simulink model "BLDC_SMC"  (R2023b)
settings: Solver=ode23tb  StartTime=0.0  StopTime=2  FixedStep=Ts  RelTol=1e-4  EnableMultiTasking=on
InitFcn:
  | Ts = 10e-6;
  | 
  | R = 2.875;
  | Ld = 8.2e-3;
  | Lq = 8.2e-3;
  | Pn = 4;
  | flux = 0.175;
model workspace (MAT data in the model file):
  LDLQ = [0.00108 0.00108]
  PN_ = 7
  RS = 4.64
  TS_1 = 0.001
undefined symbols (not defined in the file): DiscIntNeverNeededParam
libraries: simulink x14, powerlib_extras x12, spsPermanentMagnetSynchronousMachineLib x6, spsUniversalBridgeLib x6, spsDCVoltageSourceLib x6, sps_lib x6, dspindex x2, visionanalysis x1, dspstat3 x1, dspfdesign x1
(part 1 of 3)
settings Model: PacingRate=100  Creator=SUN  LastModifiedBy=Shykerboy
settings SolverCC: ZeroCrossControl=DisableAll  AlgebraicLoopSolver=TrustRegion
settings DataIOCC: LimitDataPoints=on  SaveFormat=Array  SignalLoggingSaveFormat=ModelDataLogs  ReturnWorkspaceOutputs=off
settings OptimizationCC: ExpressionDepthLimit=2147483647  InitFltsAndDblsToZero=on  LifeSpan=inf
settings DebuggingCC: UnderspecifiedInitializationDetection=Classic  MergeDetectMultiDrivingBlocksExec=none  SolverPrmCheckMsg=warning  FcnCallInpInsideContextMsg=warning  UnconnectedInputMsg=warning  UnconnectedOutputMsg=warning  UnconnectedLineMsg=warning  StateNameClashWarn=warning  SFUnexpectedBacktrackingDiag=warning  SFNoUnconditionalDefaultTransitionDiag=warning  SFExecutionAtInitializationDiag=none  ArithmeticOperatorsInVariantConditions=warning
settings HardwareCC: ProdBitPerPointer=32  ProdBitPerSizeT=32  ProdBitPerPtrDiffT=32  ProdLargestAtomicFloat=None  ProdIntDivRoundTo=Undefined  ProdEndianess=Unspecified  ProdWordSize=32  ProdHWDeviceType=32-bit Generic
settings ModelReferenceCC: PropagateSignalLabelsOutOfModel=off
settings SFSimCC: SimUseLocalCustomCode=off  CustomCodeUndefinedFunction=UseInterfaceOnly
settings RTWCC: RTWUseLocalCustomCode=off
settings CodeAppCC: StateflowObjectComments=on
settings GRTTargetCC: TargetLangStandard=C89/C90 (ANSI)  CombineOutputUpdateFcns=off  GRTInterface=on
settings ConfigComp: CovMetricSettings=dw  CovSaveCumulativeToWorkspaceVar=on  CovSaveSingleToWorkspaceVar=on  CovExternalEMLEnable=off  CovSFcnEnable=off
settings SimscapeCC: SimscapeNormalizeSystem=off

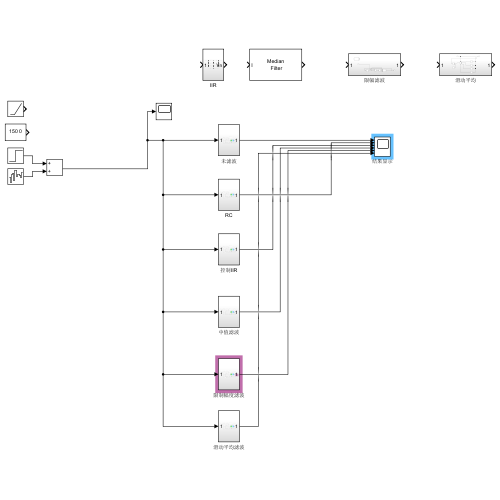
[thumbnail: Simulink's stored preview of the top-level diagram]
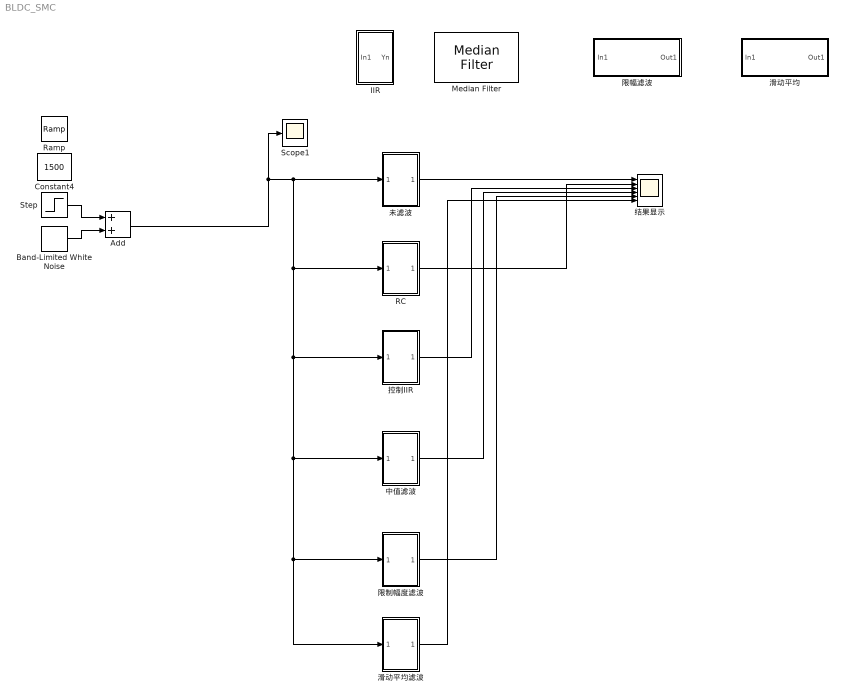
== system BLDC_SMC ==
  Add : Sum
  Band-Limited White Noise : simulink/Sources/Band-Limited White Noise  Cov=[0.100]  Ts=0.001  seed=[23341]
  Constant4 : Constant  Value=1500  SampleTime=1e-3
  IIR : Subsystem
  Median Filter : visionanalysis/Median Filter  nghbood=[3 3]  outSize=Same as input port I  padType=Constant  padSrc=Specify via dialog  padVal=0  roundingMode=Floor  overflowMode=off
  RC : Subsystem
  Ramp : simulink/Sources/Ramp  slope=500  start=0  InitialOutput=0
  Scope1 : Scope
  Step : Step  Time=0.5  After=1000  SampleTime=1e-3
  中值滤波 : Subsystem
  控制IIR : Subsystem
  未滤波 : Subsystem
  滑动平均 : Subsystem
  滑动平均滤波 : Subsystem
  结果显示 : Scope  NumInputPorts=6
  限制幅度滤波 : Subsystem
  限幅滤波 : Subsystem
  wires:
  未滤波/1(Out1) -> 结果显示/1
  Step/1 -> Add/1
  Band-Limited White Noise/1 -> Add/2
  Add/1 -> Scope1/1, 滑动平均滤波/1(In1), 限制幅度滤波/1(In1), 中值滤波/1(In1), 控制IIR/1(In1), RC/1(In1), 未滤波/1(In1)
  RC/1(Out1) -> 结果显示/2
  控制IIR/1(Out1) -> 结果显示/3
  中值滤波/1(Out1) -> 结果显示/4
  限制幅度滤波/1(Out1) -> 结果显示/5
  滑动平均滤波/1(Out1) -> 结果显示/6

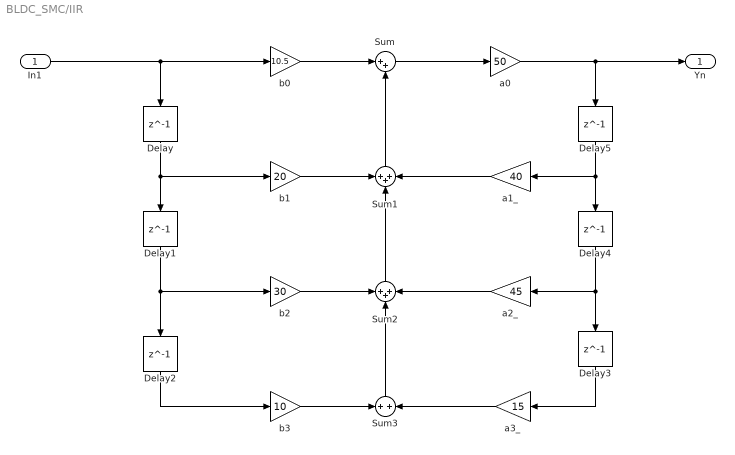
== system BLDC_SMC/IIR ==
  In1 : Inport
  Delay{,1..5} (6 alike) : Delay  DelayLength=1
  Sum : Sum  Inputs=|++
  Sum1 : Sum  Inputs=+++
  Sum2 : Sum  Inputs=+++
  Sum3 : Sum  Inputs=+|+
  a0 : Gain  Gain=50
  a1_ : Gain  Gain=40
  a2_ : Gain  Gain=45
  a3_ : Gain  Gain=15
  b0 : Gain  Gain=10.5
  b1 : Gain  Gain=20
  b2 : Gain  Gain=30
  b3 : Gain  Gain=10
  Yn : Outport
  wires:
  Delay5/1 -> a1_/1, Delay4/1
  Sum2/1 -> Sum1/2
  Delay/1 -> b1/1, Delay1/1
  a3_/1 -> Sum3/2
  Delay1/1 -> b2/1, Delay2/1
  b1/1 -> Sum1/1
  Delay3/1 -> a3_/1
  a0/1 -> Yn/1, Delay5/1
  b3/1 -> Sum3/1
  Delay4/1 -> a2_/1, Delay3/1
  b0/1 -> Sum/1
  a2_/1 -> Sum2/3
  Sum3/1 -> Sum2/2
  a1_/1 -> Sum1/3
  Sum1/1 -> Sum/2
  Delay2/1 -> b3/1
  b2/1 -> Sum2/1
  Sum/1 -> a0/1
  In1/1 -> b0/1, Delay/1

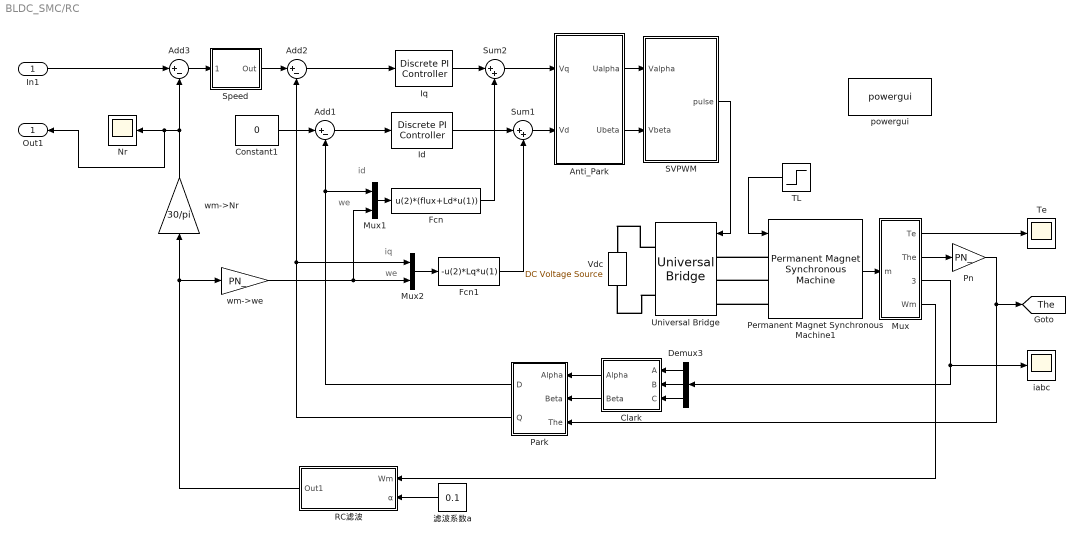
== system BLDC_SMC/RC ==
  note: iq
  note: we
  note: we
  note: id
  In1 : Inport
  Add1 : Sum  Inputs=|+-
  Add2 : Sum  Inputs=|+-
  Add3 : Sum  Inputs=|+-
  Anti_Park : Subsystem
  Clark : Subsystem
  Constant1 : Constant  Value=0
  Demux3 : Demux  Outputs=3
  Fcn : Fcn  Expr=u(2)*(flux+Ld*u(1))
  Fcn1 : Fcn  Expr=-u(2)*Lq*u(1)
  Id : powerlib_extras/Discrete  Control Blocks/Discrete PI Controller  Kp=Ld*2000  Ki=RS*2000  Par_Limits=[311*0.9*sqrt(1/3) -311*0.9*sqrt(1/3)]  Init=0  Ts=TS_1
  Iq : powerlib_extras/Discrete  Control Blocks/Discrete PI Controller  Kp=Lq*2000  Ki=RS*2000  Par_Limits=[311*0.9*sqrt(1/3) -311*0.9*sqrt(1/3)]  Init=0  Ts=TS_1
  Mux : Subsystem
  Mux1 : Mux  Inputs=2
  Mux2 : Mux  Inputs=2
  Nr : Scope
  Park : Subsystem
  Permanent Magnet Synchronous Machine1 : spsPermanentMagnetSynchronousMachineLib/Permanent Magnet Synchronous Machine  NbPhases=3  FluxDistribution=Sinusoidal  RotorType=Salient-pole  MechanicalLoad=Torque Tm  PresetModel=No  ShowDetailedParameters=on  MeasurementBus=off  Resistance=RS  Inductance=8.5e-3  dqInductances=LDLQ  La=0.000835  MachineConstant=Flux linkage established by magnets (V.s)  Flux=0.175  VoltageCst=222.1904  TorqueCst=1.8375  Flat=120  Mechanical=[0.003 0.008 7 0]  PolePairs=3  InitialConditions=[0,0, 0,0]  InitialConditions5ph=[0 0 0 0 0 0]  RefAngle=Aligned with phase A axis (original Park)  IterativeDiscreteModel=Trapezoidal non iterative  TsBlock=-1  TsPowergui=0
  Pn : Gain  Gain=PN_
  RC滤波 : Subsystem
  SVPWM : Subsystem
  Speed : Subsystem  AncestorBlock=|  DialogController=POWERSYS.PowerSysDialog  mask(Discrete PI Controller){C=60, Mu=200, q=300, Par_Limits=[30 -30], Init=0, Ts=TS_1}
      | powerlib_extras/Discrete 
      | Control Blocks/Discrete
      | PI Controller
      mask prompts: C "Gain (c):"; Mu "Gain (Mu):"; q "Gain (q)"; Par_Limits "Output limits: [ Upper   Lower ]"; Init "Output initial value:"; Ts "Sample time:"
      mask help: This block implements a discrete PI controller.
      mask init:
      | UpperLimit=Par_Limits(1);
      | LowerLimit=Par_Limits(2);
      | power_initmask();
      mask Help: This block is part of a subset of blocks in the Extras library that does not have documentation associated with it, other than the block mask description.
      mask Display: disp('SMC');
  Sum1 : Sum  Inputs=|++
  Sum2 : Sum  Inputs=|++
  TL : Step  Time=0.2  After=10  SampleTime=0
  Te : Scope
  Universal Bridge : spsUniversalBridgeLib/Universal Bridge  Arms=3  SnubberResistance=1e5  SnubberCapacitance=inf  Device=IGBT / Diodes  Ron=1e-3  Lon=0  ForwardVoltages="[  0  0  ]"  ForwardVoltage=0  GTOparameters=[ 10e-6 , 20e-6 ]  IGBTparameters=[ 1e-6 , 2e-6 ]  Measurements=None  Measurements_2=None  converterType=Rectifier
  Vdc : spsDCVoltageSourceLib/DC Voltage Source  Amplitude=311  Measurements=None
  iabc : Scope
  powergui : sps_lib/powergui  SimulationMode=Continuous  SampleTime=Ts  frequency=60  Iterations=50  frequencyindice=0  Pbase=100e6  ErrMax=1e-4  UnitsV=kV  UnitsW=MW  buscounter=0  FunctionMessages=off  echomessages=off  EnableUseOfTLC=off  CurrentSourceSwitches=on  DisableSnubberDevices=off  DisableRonSwitches=off  DisableVfSwitches=off  DisplayEquations=off  AutomaticDiscreteSolvers=off  SolverType=Tustin/Backward Euler (TBE)  Interpol=off  ExternalGateDelay=off  methode=off  Ts=0  x0status=blocks  SPID=off  SwTol=0  HookPort=off  NonlinearTolerance=1e-4  nMaxIteration=100  ContinueOnMaxIteration=off  RestoreLinks=warning  ResistiveCurrentMeasurement=off  Frange=[0:2:500]  Ylog=off  Xlog=on  ShowGrid=off  save=off  variable=ZData  structure=0  ZoomFFT=on  StartTime=0.0  cycles=1  DisplayStyle=1  fundamental=60  FreqAxis=off  MaxFrequency=1000  frequencyindicesteady=1  RmsSteady=1  display=off
  wm->Nr : Gain  Gain=30/pi
  wm->we : Gain  Gain=PN_
  滤波系数a : Constant  Value=0.1
  Out1 : Outport
  tag scope: The=global
  wires:
  Pn/1 -> Park/3(The), [The]
  SVPWM/1(pulse) -> Universal Bridge/1
  Add1/1 -> Id/1
  In1/1 -> Add3/1
  Fcn/1 -> Sum2/2
  Id/1 -> Sum1/1
  Mux2/1 -> Fcn1/1
  wm->Nr/1 -> Add3/2, Out1/1, Nr/1
  Clark/2(Beta) -> Park/2(Beta)
  Iq/1 -> Sum2/1
  Sum2/1 -> Anti_Park/1(Vq)
  Speed/1(Out) -> Add2/1
  Add2/1 -> Iq/1
  Fcn1/1 -> Sum1/2
  Park/2(Q) -> Mux2/1, Add2/2
  Constant1/1 -> Add1/1
  Sum1/1 -> Anti_Park/2(Vd)
  Add3/1 -> Speed/1(Error)
  Mux/1(Te) -> Te/1
  Mux/2(The) -> Pn/1
  Anti_Park/2(Ubeta) -> SVPWM/2(Vbeta)
  Demux3/1 -> Clark/1(A)
  Demux3/3 -> Clark/3(C)
  Mux/3(Iabc) -> iabc/1, Demux3/1
  Demux3/2 -> Clark/2(B)
  Mux1/1 -> Fcn/1
  TL/1 -> Permanent Magnet Synchronous Machine1/1
  Permanent Magnet Synchronous Machine1/1 -> Mux/1(m)
  Clark/1(Alpha) -> Park/1(Alpha)
  Park/1(D) -> Mux1/1, Add1/2
  Anti_Park/1(Ualpha) -> SVPWM/1(Valpha)
  wm->we/1 -> Mux2/2, Mux1/2
  Mux/4(Wm) -> RC滤波/1(Wm)
  滤波系数a/1 -> RC滤波/2(α)
  RC滤波/1(Out1) -> wm->we/1, wm->Nr/1
  connections:
  Permanent Magnet Synchronous Machine1/LConn2 -- Universal Bridge/LConn2
  Universal Bridge/RConn1 -- Vdc/RConn1
  Permanent Magnet Synchronous Machine1/LConn1 -- Universal Bridge/LConn1
  Permanent Magnet Synchronous Machine1/LConn3 -- Universal Bridge/LConn3
  Universal Bridge/RConn2 -- Vdc/LConn1

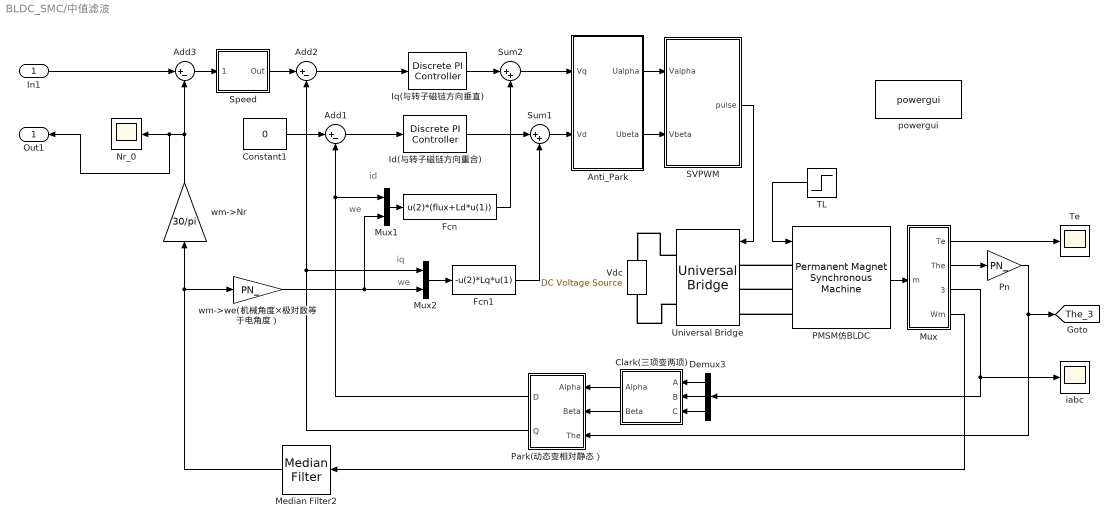
== system BLDC_SMC/中值滤波 ==
  note: iq
  note: we
  note: we
  note: id
  In1 : Inport
  Add1 : Sum  Inputs=|+-
  Add2 : Sum  Inputs=|+-
  Add3 : Sum  Inputs=|+-
  Anti_Park : Subsystem
  Clark(三项变两项) : Subsystem
  Constant1 : Constant  Value=0
  Demux3 : Demux  Outputs=3
  Fcn : Fcn  Expr=u(2)*(flux+Ld*u(1))
  Fcn1 : Fcn  Expr=-u(2)*Lq*u(1)
  Id(与转子磁链方向重合) : powerlib_extras/Discrete  Control Blocks/Discrete PI Controller  Kp=Ld*2000  Ki=RS*2000  Par_Limits=[311*0.9*sqrt(1/3) -311*0.9*sqrt(1/3)]  Init=0  Ts=TS_1
  Iq(与转子磁链方向垂直) : powerlib_extras/Discrete  Control Blocks/Discrete PI Controller  Kp=Lq*2000  Ki=RS*2000  Par_Limits=[311*0.9*sqrt(1/3) -311*0.9*sqrt(1/3)]  Init=0  Ts=TS_1
  Median Filter2 : dspstat3/Median Filter  WindowLength=5  SimulateUsing=Code generation
  Mux : Subsystem
  Mux1 : Mux  Inputs=2
  Mux2 : Mux  Inputs=2
  Nr_0 : Scope
  PMSM仿BLDC : spsPermanentMagnetSynchronousMachineLib/Permanent Magnet Synchronous Machine  NbPhases=3  FluxDistribution=Sinusoidal  RotorType=Salient-pole  MechanicalLoad=Torque Tm  PresetModel=No  ShowDetailedParameters=on  MeasurementBus=off  Resistance=RS  Inductance=8.5e-3  dqInductances=LDLQ  La=0.000835  MachineConstant=Flux linkage established by magnets (V.s)  Flux=0.175  VoltageCst=222.1904  TorqueCst=1.8375  Flat=120  Mechanical=[0.003 0.008 7 0]  PolePairs=3  InitialConditions=[0,0, 0,0]  InitialConditions5ph=[0 0 0 0 0 0]  RefAngle=Aligned with phase A axis (original Park)  IterativeDiscreteModel=Trapezoidal non iterative  TsBlock=-1  TsPowergui=0
  Park(动态变相对静态） : Subsystem
  Pn : Gain  Gain=PN_
  SVPWM : Subsystem
  Speed : Subsystem  AncestorBlock=|  DialogController=POWERSYS.PowerSysDialog  mask(Discrete PI Controller){C=60, Mu=200, q=300, Par_Limits=[30 -30], Init=0, Ts=TS_1}
      | powerlib_extras/Discrete 
      | Control Blocks/Discrete
      | PI Controller
      mask prompts: C "Gain (c):"; Mu "Gain (Mu):"; q "Gain (q)"; Par_Limits "Output limits: [ Upper   Lower ]"; Init "Output initial value:"; Ts "Sample time:"
      mask help: This block implements a discrete PI controller.
      mask init:
      | UpperLimit=Par_Limits(1);
      | LowerLimit=Par_Limits(2);
      | power_initmask();
      mask Help: This block is part of a subset of blocks in the Extras library that does not have documentation associated with it, other than the block mask description.
      mask Display: disp('SMC');
  Sum1 : Sum  Inputs=|++
  Sum2 : Sum  Inputs=|++
  TL : Step  Time=0.2  After=10  SampleTime=0
  Te : Scope
  Universal Bridge : spsUniversalBridgeLib/Universal Bridge  Arms=3  SnubberResistance=1e5  SnubberCapacitance=inf  Device=IGBT / Diodes  Ron=1e-3  Lon=0  ForwardVoltages="[  0  0  ]"  ForwardVoltage=0  GTOparameters=[ 10e-6 , 20e-6 ]  IGBTparameters=[ 1e-6 , 2e-6 ]  Measurements=None  Measurements_2=None  converterType=Rectifier
  Vdc : spsDCVoltageSourceLib/DC Voltage Source  Amplitude=311  Measurements=None
  iabc : Scope
  powergui : sps_lib/powergui  SimulationMode=Continuous  SampleTime=Ts  frequency=60  Iterations=50  frequencyindice=0  Pbase=100e6  ErrMax=1e-4  UnitsV=kV  UnitsW=MW  buscounter=0  FunctionMessages=off  echomessages=off  EnableUseOfTLC=off  CurrentSourceSwitches=on  DisableSnubberDevices=off  DisableRonSwitches=off  DisableVfSwitches=off  DisplayEquations=off  AutomaticDiscreteSolvers=off  SolverType=Tustin/Backward Euler (TBE)  Interpol=off  ExternalGateDelay=off  methode=off  Ts=0  x0status=blocks  SPID=off  SwTol=0  HookPort=off  NonlinearTolerance=1e-4  nMaxIteration=100  ContinueOnMaxIteration=off  RestoreLinks=warning  ResistiveCurrentMeasurement=off  Frange=[0:2:500]  Ylog=off  Xlog=on  ShowGrid=off  save=off  variable=ZData  structure=0  ZoomFFT=on  StartTime=0.0  cycles=1  DisplayStyle=1  fundamental=60  FreqAxis=off  MaxFrequency=1000  frequencyindicesteady=1  RmsSteady=1  display=off
  wm->Nr : Gain  Gain=30/pi
  wm->we(机械角度×极对数等于电角度） : Gain  Gain=PN_
  Out1 : Outport
  tag scope: The_3=global
  wires:
  Pn/1 -> Park(动态变相对静态）/3(The), [The_3]
  SVPWM/1(pulse) -> Universal Bridge/1
  Add1/1 -> Id(与转子磁链方向重合)/1
  In1/1 -> Add3/1
  Fcn/1 -> Sum2/2
  Id(与转子磁链方向重合)/1 -> Sum1/1
  Mux2/1 -> Fcn1/1
  wm->Nr/1 -> Add3/2, Out1/1, Nr_0/1
  Clark(三项变两项)/2(Beta) -> Park(动态变相对静态）/2(Beta)
  Iq(与转子磁链方向垂直)/1 -> Sum2/1
  Sum2/1 -> Anti_Park/1(Vq)
  Speed/1(Out) -> Add2/1
  Add2/1 -> Iq(与转子磁链方向垂直)/1
  Fcn1/1 -> Sum1/2
  Park(动态变相对静态）/2(Q) -> Mux2/1, Add2/2
  Constant1/1 -> Add1/1
  Sum1/1 -> Anti_Park/2(Vd)
  Add3/1 -> Speed/1(Error)
  Mux/1(Te) -> Te/1
  Mux/2(The) -> Pn/1
  Anti_Park/2(Ubeta) -> SVPWM/2(Vbeta)
  Demux3/1 -> Clark(三项变两项)/1(A)
  Demux3/3 -> Clark(三项变两项)/3(C)
  Mux/3(Iabc) -> iabc/1, Demux3/1
  Demux3/2 -> Clark(三项变两项)/2(B)
  Mux1/1 -> Fcn/1
  TL/1 -> PMSM仿BLDC/1
  PMSM仿BLDC/1 -> Mux/1(m)
  Clark(三项变两项)/1(Alpha) -> Park(动态变相对静态）/1(Alpha)
  Park(动态变相对静态）/1(D) -> Mux1/1, Add1/2
  Anti_Park/1(Ualpha) -> SVPWM/1(Valpha)
  wm->we(机械角度×极对数等于电角度）/1 -> Mux2/2, Mux1/2
  Mux/4(Wm) -> Median Filter2/1
  Median Filter2/1 -> wm->Nr/1, wm->we(机械角度×极对数等于电角度）/1
  connections:
  PMSM仿BLDC/LConn2 -- Universal Bridge/LConn2
  Universal Bridge/RConn1 -- Vdc/RConn1
  PMSM仿BLDC/LConn1 -- Universal Bridge/LConn1
  PMSM仿BLDC/LConn3 -- Universal Bridge/LConn3
  Universal Bridge/RConn2 -- Vdc/LConn1

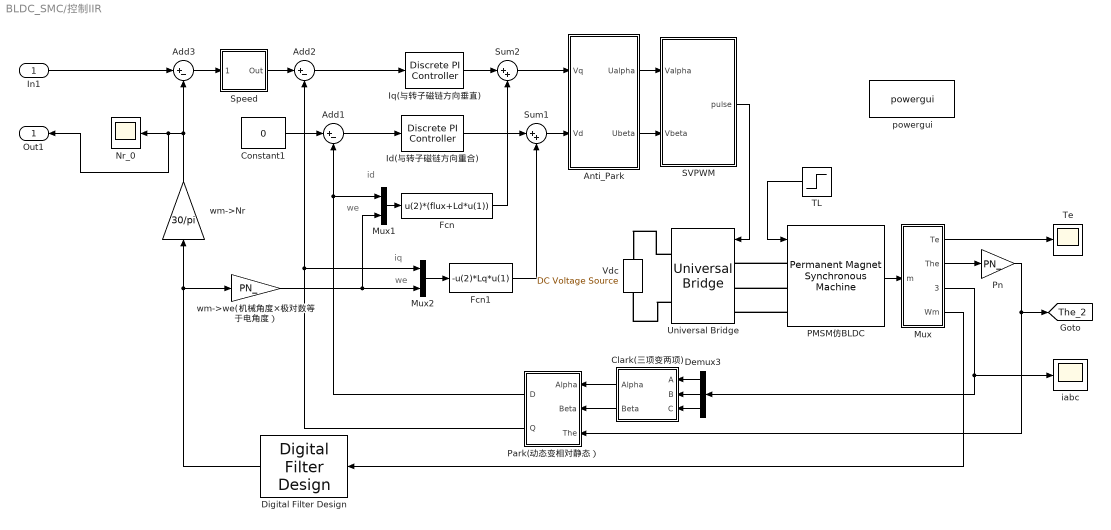
== system BLDC_SMC/控制IIR ==
  note: iq
  note: we
  note: we
  note: id
  In1 : Inport
  Add1 : Sum  Inputs=|+-
  Add2 : Sum  Inputs=|+-
  Add3 : Sum  Inputs=|+-
  Anti_Park : Subsystem
  Clark(三项变两项) : Subsystem
  Constant1 : Constant  Value=0
  Demux3 : Demux  Outputs=3
  Digital Filter Design : dspfdesign/Digital Filter Design  mwdsp_browser_bugfix_var=off
  Fcn : Fcn  Expr=u(2)*(flux+Ld*u(1))
  Fcn1 : Fcn  Expr=-u(2)*Lq*u(1)
  Id(与转子磁链方向重合) : powerlib_extras/Discrete  Control Blocks/Discrete PI Controller  Kp=Ld*2000  Ki=RS*2000  Par_Limits=[311*0.9*sqrt(1/3) -311*0.9*sqrt(1/3)]  Init=0  Ts=TS_1
  Iq(与转子磁链方向垂直) : powerlib_extras/Discrete  Control Blocks/Discrete PI Controller  Kp=Lq*2000  Ki=RS*2000  Par_Limits=[311*0.9*sqrt(1/3) -311*0.9*sqrt(1/3)]  Init=0  Ts=TS_1
  Mux : Subsystem
  Mux1 : Mux  Inputs=2
  Mux2 : Mux  Inputs=2
  Nr_0 : Scope
  PMSM仿BLDC : spsPermanentMagnetSynchronousMachineLib/Permanent Magnet Synchronous Machine  NbPhases=3  FluxDistribution=Sinusoidal  RotorType=Salient-pole  MechanicalLoad=Torque Tm  PresetModel=No  ShowDetailedParameters=on  MeasurementBus=off  Resistance=RS  Inductance=8.5e-3  dqInductances=LDLQ  La=0.000835  MachineConstant=Flux linkage established by magnets (V.s)  Flux=0.175  VoltageCst=222.1904  TorqueCst=1.8375  Flat=120  Mechanical=[0.003 0.008 7 0]  PolePairs=3  InitialConditions=[0,0, 0,0]  InitialConditions5ph=[0 0 0 0 0 0]  RefAngle=Aligned with phase A axis (original Park)  IterativeDiscreteModel=Trapezoidal non iterative  TsBlock=-1  TsPowergui=0
  Park(动态变相对静态） : Subsystem
  Pn : Gain  Gain=PN_
  SVPWM : Subsystem
  Speed : Subsystem  AncestorBlock=|  DialogController=POWERSYS.PowerSysDialog  mask(Discrete PI Controller){C=60, Mu=200, q=300, Par_Limits=[30 -30], Init=0, Ts=TS_1}
      | powerlib_extras/Discrete 
      | Control Blocks/Discrete
      | PI Controller
      mask prompts: C "Gain (c):"; Mu "Gain (Mu):"; q "Gain (q)"; Par_Limits "Output limits: [ Upper   Lower ]"; Init "Output initial value:"; Ts "Sample time:"
      mask help: This block implements a discrete PI controller.
      mask init:
      | UpperLimit=Par_Limits(1);
      | LowerLimit=Par_Limits(2);
      | power_initmask();
      mask Help: This block is part of a subset of blocks in the Extras library that does not have documentation associated with it, other than the block mask description.
      mask Display: disp('SMC');
  Sum1 : Sum  Inputs=|++
  Sum2 : Sum  Inputs=|++
  TL : Step  Time=0.2  After=10  SampleTime=0
  Te : Scope
  Universal Bridge : spsUniversalBridgeLib/Universal Bridge  Arms=3  SnubberResistance=1e5  SnubberCapacitance=inf  Device=IGBT / Diodes  Ron=1e-3  Lon=0  ForwardVoltages="[  0  0  ]"  ForwardVoltage=0  GTOparameters=[ 10e-6 , 20e-6 ]  IGBTparameters=[ 1e-6 , 2e-6 ]  Measurements=None  Measurements_2=None  converterType=Rectifier
  Vdc : spsDCVoltageSourceLib/DC Voltage Source  Amplitude=311  Measurements=None
  iabc : Scope
  powergui : sps_lib/powergui  SimulationMode=Continuous  SampleTime=Ts  frequency=60  Iterations=50  frequencyindice=0  Pbase=100e6  ErrMax=1e-4  UnitsV=kV  UnitsW=MW  buscounter=0  FunctionMessages=off  echomessages=off  EnableUseOfTLC=off  CurrentSourceSwitches=on  DisableSnubberDevices=off  DisableRonSwitches=off  DisableVfSwitches=off  DisplayEquations=off  AutomaticDiscreteSolvers=off  SolverType=Tustin/Backward Euler (TBE)  Interpol=off  ExternalGateDelay=off  methode=off  Ts=0  x0status=blocks  SPID=off  SwTol=0  HookPort=off  NonlinearTolerance=1e-4  nMaxIteration=100  ContinueOnMaxIteration=off  RestoreLinks=warning  ResistiveCurrentMeasurement=off  Frange=[0:2:500]  Ylog=off  Xlog=on  ShowGrid=off  save=off  variable=ZData  structure=0  ZoomFFT=on  StartTime=0.0  cycles=1  DisplayStyle=1  fundamental=60  FreqAxis=off  MaxFrequency=1000  frequencyindicesteady=1  RmsSteady=1  display=off
  wm->Nr : Gain  Gain=30/pi
  wm->we(机械角度×极对数等于电角度） : Gain  Gain=PN_
  Out1 : Outport
  tag scope: The_2=global
  wires:
  Pn/1 -> Park(动态变相对静态）/3(The), [The_2]
  SVPWM/1(pulse) -> Universal Bridge/1
  Add1/1 -> Id(与转子磁链方向重合)/1
  In1/1 -> Add3/1
  Fcn/1 -> Sum2/2
  Id(与转子磁链方向重合)/1 -> Sum1/1
  Mux2/1 -> Fcn1/1
  wm->Nr/1 -> Add3/2, Out1/1, Nr_0/1
  Clark(三项变两项)/2(Beta) -> Park(动态变相对静态）/2(Beta)
  Iq(与转子磁链方向垂直)/1 -> Sum2/1
  Sum2/1 -> Anti_Park/1(Vq)
  Speed/1(Out) -> Add2/1
  Add2/1 -> Iq(与转子磁链方向垂直)/1
  Fcn1/1 -> Sum1/2
  Park(动态变相对静态）/2(Q) -> Mux2/1, Add2/2
  Mux/4(Wm) -> Digital Filter Design/1
  Constant1/1 -> Add1/1
  Sum1/1 -> Anti_Park/2(Vd)
  Add3/1 -> Speed/1(Error)
  Mux/1(Te) -> Te/1
  Mux/2(The) -> Pn/1
  Anti_Park/2(Ubeta) -> SVPWM/2(Vbeta)
  Demux3/1 -> Clark(三项变两项)/1(A)
  Demux3/3 -> Clark(三项变两项)/3(C)
  Mux/3(Iabc) -> iabc/1, Demux3/1
  Demux3/2 -> Clark(三项变两项)/2(B)
  Mux1/1 -> Fcn/1
  TL/1 -> PMSM仿BLDC/1
  PMSM仿BLDC/1 -> Mux/1(m)
  Clark(三项变两项)/1(Alpha) -> Park(动态变相对静态）/1(Alpha)
  Park(动态变相对静态）/1(D) -> Mux1/1, Add1/2
  Anti_Park/1(Ualpha) -> SVPWM/1(Valpha)
  wm->we(机械角度×极对数等于电角度）/1 -> Mux2/2, Mux1/2
  Digital Filter Design/1 -> wm->we(机械角度×极对数等于电角度）/1, wm->Nr/1
  connections:
  PMSM仿BLDC/LConn2 -- Universal Bridge/LConn2
  Universal Bridge/RConn1 -- Vdc/RConn1
  PMSM仿BLDC/LConn1 -- Universal Bridge/LConn1
  PMSM仿BLDC/LConn3 -- Universal Bridge/LConn3
  Universal Bridge/RConn2 -- Vdc/LConn1

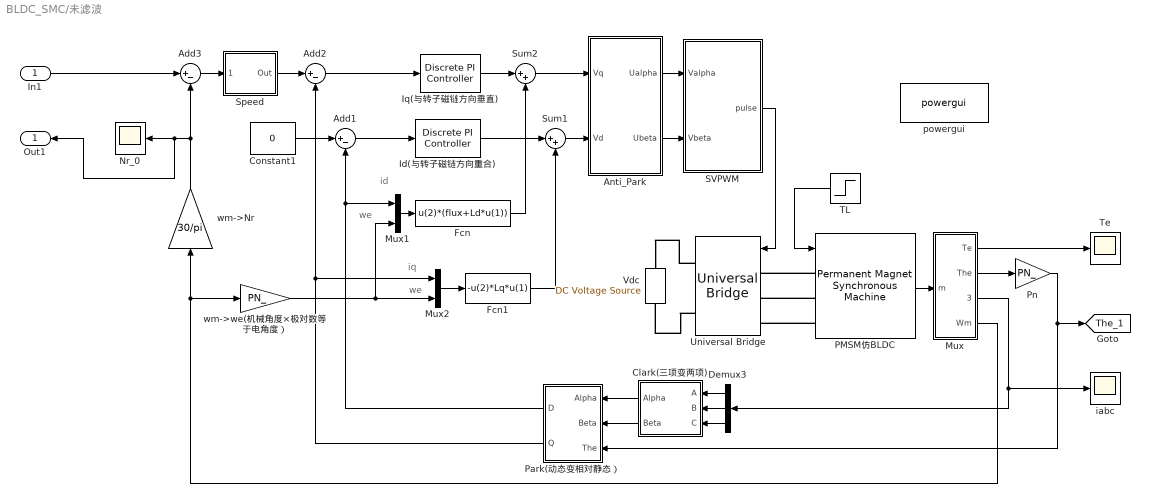
== system BLDC_SMC/未滤波 ==
  note: iq
  note: we
  note: we
  note: id
  In1 : Inport
  Add1 : Sum  Inputs=|+-
  Add2 : Sum  Inputs=|+-
  Add3 : Sum  Inputs=|+-
  Anti_Park : Subsystem
  Clark(三项变两项) : Subsystem
  Constant1 : Constant  Value=0
  Demux3 : Demux  Outputs=3
  Fcn : Fcn  Expr=u(2)*(flux+Ld*u(1))
  Fcn1 : Fcn  Expr=-u(2)*Lq*u(1)
  Id(与转子磁链方向重合) : powerlib_extras/Discrete  Control Blocks/Discrete PI Controller  Kp=Ld*2000  Ki=RS*2000  Par_Limits=[311*0.9*sqrt(1/3) -311*0.9*sqrt(1/3)]  Init=0  Ts=TS_1
  Iq(与转子磁链方向垂直) : powerlib_extras/Discrete  Control Blocks/Discrete PI Controller  Kp=Lq*2000  Ki=RS*2000  Par_Limits=[311*0.9*sqrt(1/3) -311*0.9*sqrt(1/3)]  Init=0  Ts=TS_1
  Mux : Subsystem
  Mux1 : Mux  Inputs=2
  Mux2 : Mux  Inputs=2
  Nr_0 : Scope
  PMSM仿BLDC : spsPermanentMagnetSynchronousMachineLib/Permanent Magnet Synchronous Machine  NbPhases=3  FluxDistribution=Sinusoidal  RotorType=Salient-pole  MechanicalLoad=Torque Tm  PresetModel=No  ShowDetailedParameters=on  MeasurementBus=off  Resistance=RS  Inductance=8.5e-3  dqInductances=LDLQ  La=0.000835  MachineConstant=Flux linkage established by magnets (V.s)  Flux=0.175  VoltageCst=222.1904  TorqueCst=1.8375  Flat=120  Mechanical=[0.003 0.008 7 0]  PolePairs=3  InitialConditions=[0,0, 0,0]  InitialConditions5ph=[0 0 0 0 0 0]  RefAngle=Aligned with phase A axis (original Park)  IterativeDiscreteModel=Trapezoidal non iterative  TsBlock=-1  TsPowergui=0
  Park(动态变相对静态） : Subsystem
  Pn : Gain  Gain=PN_
  SVPWM : Subsystem
  Speed : Subsystem  AncestorBlock=|  DialogController=POWERSYS.PowerSysDialog  mask(Discrete PI Controller){C=60, Mu=200, q=300, Par_Limits=[30 -30], Init=0, Ts=TS_1}
      | powerlib_extras/Discrete 
      | Control Blocks/Discrete
      | PI Controller
      mask prompts: C "Gain (c):"; Mu "Gain (Mu):"; q "Gain (q)"; Par_Limits "Output limits: [ Upper   Lower ]"; Init "Output initial value:"; Ts "Sample time:"
      mask help: This block implements a discrete PI controller.
      mask init:
      | UpperLimit=Par_Limits(1);
      | LowerLimit=Par_Limits(2);
      | power_initmask();
      mask Help: This block is part of a subset of blocks in the Extras library that does not have documentation associated with it, other than the block mask description.
      mask Display: disp('SMC');
  Sum1 : Sum  Inputs=|++
  Sum2 : Sum  Inputs=|++
  TL : Step  Time=0.2  After=10  SampleTime=0
  Te : Scope
  Universal Bridge : spsUniversalBridgeLib/Universal Bridge  Arms=3  SnubberResistance=1e5  SnubberCapacitance=inf  Device=IGBT / Diodes  Ron=1e-3  Lon=0  ForwardVoltages="[  0  0  ]"  ForwardVoltage=0  GTOparameters=[ 10e-6 , 20e-6 ]  IGBTparameters=[ 1e-6 , 2e-6 ]  Measurements=None  Measurements_2=None  converterType=Rectifier
  Vdc : spsDCVoltageSourceLib/DC Voltage Source  Amplitude=311  Measurements=None
  iabc : Scope
  powergui : sps_lib/powergui  SimulationMode=Continuous  SampleTime=Ts  frequency=60  Iterations=50  frequencyindice=0  Pbase=100e6  ErrMax=1e-4  UnitsV=kV  UnitsW=MW  buscounter=0  FunctionMessages=off  echomessages=off  EnableUseOfTLC=off  CurrentSourceSwitches=on  DisableSnubberDevices=off  DisableRonSwitches=off  DisableVfSwitches=off  DisplayEquations=off  AutomaticDiscreteSolvers=off  SolverType=Tustin/Backward Euler (TBE)  Interpol=off  ExternalGateDelay=off  methode=off  Ts=0  x0status=blocks  SPID=off  SwTol=0  HookPort=off  NonlinearTolerance=1e-4  nMaxIteration=100  ContinueOnMaxIteration=off  RestoreLinks=warning  ResistiveCurrentMeasurement=off  Frange=[0:2:500]  Ylog=off  Xlog=on  ShowGrid=off  save=off  variable=ZData  structure=0  ZoomFFT=on  StartTime=0.0  cycles=1  DisplayStyle=1  fundamental=60  FreqAxis=off  MaxFrequency=1000  frequencyindicesteady=1  RmsSteady=1  display=off
  wm->Nr : Gain  Gain=30/pi
  wm->we(机械角度×极对数等于电角度） : Gain  Gain=PN_
  Out1 : Outport
  tag scope: The_1=global
  wires:
  Pn/1 -> Park(动态变相对静态）/3(The), [The_1]
  SVPWM/1(pulse) -> Universal Bridge/1
  Add1/1 -> Id(与转子磁链方向重合)/1
  In1/1 -> Add3/1
  Fcn/1 -> Sum2/2
  Id(与转子磁链方向重合)/1 -> Sum1/1
  Mux2/1 -> Fcn1/1
  wm->Nr/1 -> Add3/2, Out1/1, Nr_0/1
  Clark(三项变两项)/2(Beta) -> Park(动态变相对静态）/2(Beta)
  Iq(与转子磁链方向垂直)/1 -> Sum2/1
  Sum2/1 -> Anti_Park/1(Vq)
  Speed/1(Out) -> Add2/1
  Add2/1 -> Iq(与转子磁链方向垂直)/1
  Fcn1/1 -> Sum1/2
  Park(动态变相对静态）/2(Q) -> Mux2/1, Add2/2
  Mux/4(Wm) -> wm->we(机械角度×极对数等于电角度）/1, wm->Nr/1
  Constant1/1 -> Add1/1
  Sum1/1 -> Anti_Park/2(Vd)
  Add3/1 -> Speed/1(Error)
  Mux/1(Te) -> Te/1
  Mux/2(The) -> Pn/1
  Anti_Park/2(Ubeta) -> SVPWM/2(Vbeta)
  Demux3/1 -> Clark(三项变两项)/1(A)
  Demux3/3 -> Clark(三项变两项)/3(C)
  Mux/3(Iabc) -> iabc/1, Demux3/1
  Demux3/2 -> Clark(三项变两项)/2(B)
  Mux1/1 -> Fcn/1
  TL/1 -> PMSM仿BLDC/1
  PMSM仿BLDC/1 -> Mux/1(m)
  Clark(三项变两项)/1(Alpha) -> Park(动态变相对静态）/1(Alpha)
  Park(动态变相对静态）/1(D) -> Mux1/1, Add1/2
  Anti_Park/1(Ualpha) -> SVPWM/1(Valpha)
  wm->we(机械角度×极对数等于电角度）/1 -> Mux2/2, Mux1/2
  connections:
  PMSM仿BLDC/LConn2 -- Universal Bridge/LConn2
  Universal Bridge/RConn1 -- Vdc/RConn1
  PMSM仿BLDC/LConn1 -- Universal Bridge/LConn1
  PMSM仿BLDC/LConn3 -- Universal Bridge/LConn3
  Universal Bridge/RConn2 -- Vdc/LConn1

== system BLDC_SMC/滑动平均 ==
  In1 : Inport
  Add : Sum  Inputs=+++++
  Constant : Constant  Value=5
  Delay : Delay  DelayLength=1  InitialCondition=0
  Delay1 : Delay  InitialCondition=0
  Delay2 : Delay  DelayLength=3  InitialCondition=0
  Delay3 : Delay  DelayLength=4  InitialCondition=0
  Product : Product  Inputs=*/
  Out1 : Outport
  wires:
  In1/1 -> Add/1, Delay3/1, Delay2/1, Delay1/1, Delay/1
  Delay/1 -> Add/2
  Delay1/1 -> Add/3
  Delay2/1 -> Add/4
  Delay3/1 -> Add/5
  Add/1 -> Product/1
  Constant/1 -> Product/2
  Product/1 -> Out1/1

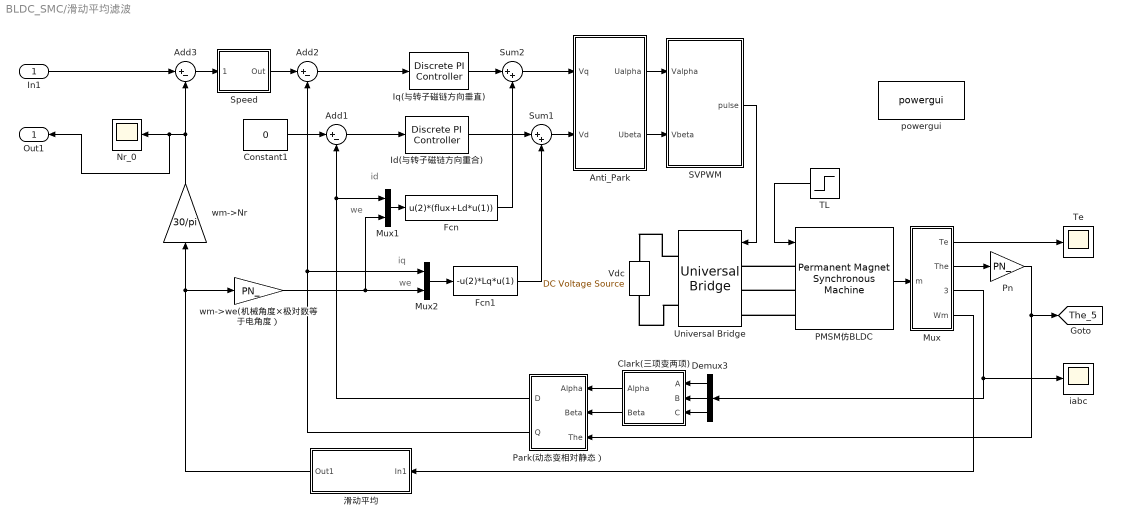
== system BLDC_SMC/滑动平均滤波 ==
  note: iq
  note: we
  note: we
  note: id
  In1 : Inport
  Add1 : Sum  Inputs=|+-
  Add2 : Sum  Inputs=|+-
  Add3 : Sum  Inputs=|+-
  Anti_Park : Subsystem
  Clark(三项变两项) : Subsystem
  Constant1 : Constant  Value=0
  Demux3 : Demux  Outputs=3
  Fcn : Fcn  Expr=u(2)*(flux+Ld*u(1))
  Fcn1 : Fcn  Expr=-u(2)*Lq*u(1)
  Id(与转子磁链方向重合) : powerlib_extras/Discrete  Control Blocks/Discrete PI Controller  Kp=Ld*2000  Ki=RS*2000  Par_Limits=[311*0.9*sqrt(1/3) -311*0.9*sqrt(1/3)]  Init=0  Ts=TS_1
  Iq(与转子磁链方向垂直) : powerlib_extras/Discrete  Control Blocks/Discrete PI Controller  Kp=Lq*2000  Ki=RS*2000  Par_Limits=[311*0.9*sqrt(1/3) -311*0.9*sqrt(1/3)]  Init=0  Ts=TS_1
  Mux : Subsystem
  Mux1 : Mux  Inputs=2
  Mux2 : Mux  Inputs=2
  Nr_0 : Scope
  PMSM仿BLDC : spsPermanentMagnetSynchronousMachineLib/Permanent Magnet Synchronous Machine  NbPhases=3  FluxDistribution=Sinusoidal  RotorType=Salient-pole  MechanicalLoad=Torque Tm  PresetModel=No  ShowDetailedParameters=on  MeasurementBus=off  Resistance=RS  Inductance=8.5e-3  dqInductances=LDLQ  La=0.000835  MachineConstant=Flux linkage established by magnets (V.s)  Flux=0.175  VoltageCst=222.1904  TorqueCst=1.8375  Flat=120  Mechanical=[0.003 0.008 7 0]  PolePairs=3  InitialConditions=[0,0, 0,0]  InitialConditions5ph=[0 0 0 0 0 0]  RefAngle=Aligned with phase A axis (original Park)  IterativeDiscreteModel=Trapezoidal non iterative  TsBlock=-1  TsPowergui=0
  Park(动态变相对静态） : Subsystem
  Pn : Gain  Gain=PN_
  SVPWM : Subsystem
  Speed : Subsystem  AncestorBlock=|  DialogController=POWERSYS.PowerSysDialog  mask(Discrete PI Controller){C=60, Mu=200, q=300, Par_Limits=[30 -30], Init=0, Ts=TS_1}
      | powerlib_extras/Discrete 
      | Control Blocks/Discrete
      | PI Controller
      mask prompts: C "Gain (c):"; Mu "Gain (Mu):"; q "Gain (q)"; Par_Limits "Output limits: [ Upper   Lower ]"; Init "Output initial value:"; Ts "Sample time:"
      mask help: This block implements a discrete PI controller.
      mask init:
      | UpperLimit=Par_Limits(1);
      | LowerLimit=Par_Limits(2);
      | power_initmask();
      mask Help: This block is part of a subset of blocks in the Extras library that does not have documentation associated with it, other than the block mask description.
      mask Display: disp('SMC');
  Sum1 : Sum  Inputs=|++
  Sum2 : Sum  Inputs=|++
  TL : Step  Time=0.2  After=10  SampleTime=0
  Te : Scope
  Universal Bridge : spsUniversalBridgeLib/Universal Bridge  Arms=3  SnubberResistance=1e5  SnubberCapacitance=inf  Device=IGBT / Diodes  Ron=1e-3  Lon=0  ForwardVoltages="[  0  0  ]"  ForwardVoltage=0  GTOparameters=[ 10e-6 , 20e-6 ]  IGBTparameters=[ 1e-6 , 2e-6 ]  Measurements=None  Measurements_2=None  converterType=Rectifier
  Vdc : spsDCVoltageSourceLib/DC Voltage Source  Amplitude=311  Measurements=None
  iabc : Scope
  powergui : sps_lib/powergui  SimulationMode=Continuous  SampleTime=Ts  frequency=60  Iterations=50  frequencyindice=0  Pbase=100e6  ErrMax=1e-4  UnitsV=kV  UnitsW=MW  buscounter=0  FunctionMessages=off  echomessages=off  EnableUseOfTLC=off  CurrentSourceSwitches=on  DisableSnubberDevices=off  DisableRonSwitches=off  DisableVfSwitches=off  DisplayEquations=off  AutomaticDiscreteSolvers=off  SolverType=Tustin/Backward Euler (TBE)  Interpol=off  ExternalGateDelay=off  methode=off  Ts=0  x0status=blocks  SPID=off  SwTol=0  HookPort=off  NonlinearTolerance=1e-4  nMaxIteration=100  ContinueOnMaxIteration=off  RestoreLinks=warning  ResistiveCurrentMeasurement=off  Frange=[0:2:500]  Ylog=off  Xlog=on  ShowGrid=off  save=off  variable=ZData  structure=0  ZoomFFT=on  StartTime=0.0  cycles=1  DisplayStyle=1  fundamental=60  FreqAxis=off  MaxFrequency=1000  frequencyindicesteady=1  RmsSteady=1  display=off
  wm->Nr : Gain  Gain=30/pi
  wm->we(机械角度×极对数等于电角度） : Gain  Gain=PN_
  滑动平均 : Subsystem
  Out1 : Outport
  tag scope: The_5=global
  wires:
  Pn/1 -> Park(动态变相对静态）/3(The), [The_5]
  SVPWM/1(pulse) -> Universal Bridge/1
  Add1/1 -> Id(与转子磁链方向重合)/1
  In1/1 -> Add3/1
  Fcn/1 -> Sum2/2
  Id(与转子磁链方向重合)/1 -> Sum1/1
  Mux2/1 -> Fcn1/1
  wm->Nr/1 -> Add3/2, Out1/1, Nr_0/1
  Clark(三项变两项)/2(Beta) -> Park(动态变相对静态）/2(Beta)
  Iq(与转子磁链方向垂直)/1 -> Sum2/1
  Sum2/1 -> Anti_Park/1(Vq)
  Speed/1(Out) -> Add2/1
  Add2/1 -> Iq(与转子磁链方向垂直)/1
  Fcn1/1 -> Sum1/2
  Park(动态变相对静态）/2(Q) -> Mux2/1, Add2/2
  Mux/4(Wm) -> 滑动平均/1(In1)
  Constant1/1 -> Add1/1
  Sum1/1 -> Anti_Park/2(Vd)
  Add3/1 -> Speed/1(Error)
  Mux/1(Te) -> Te/1
  Mux/2(The) -> Pn/1
  Anti_Park/2(Ubeta) -> SVPWM/2(Vbeta)
  Demux3/1 -> Clark(三项变两项)/1(A)
  Demux3/3 -> Clark(三项变两项)/3(C)
  Mux/3(Iabc) -> iabc/1, Demux3/1
  Demux3/2 -> Clark(三项变两项)/2(B)
  Mux1/1 -> Fcn/1
  TL/1 -> PMSM仿BLDC/1
  PMSM仿BLDC/1 -> Mux/1(m)
  Clark(三项变两项)/1(Alpha) -> Park(动态变相对静态）/1(Alpha)
  Park(动态变相对静态）/1(D) -> Mux1/1, Add1/2
  Anti_Park/1(Ualpha) -> SVPWM/1(Valpha)
  wm->we(机械角度×极对数等于电角度）/1 -> Mux2/2, Mux1/2
  滑动平均/1(Out1) -> wm->we(机械角度×极对数等于电角度）/1, wm->Nr/1
  connections:
  PMSM仿BLDC/LConn2 -- Universal Bridge/LConn2
  Universal Bridge/RConn1 -- Vdc/RConn1
  PMSM仿BLDC/LConn1 -- Universal Bridge/LConn1
  PMSM仿BLDC/LConn3 -- Universal Bridge/LConn3
  Universal Bridge/RConn2 -- Vdc/LConn1

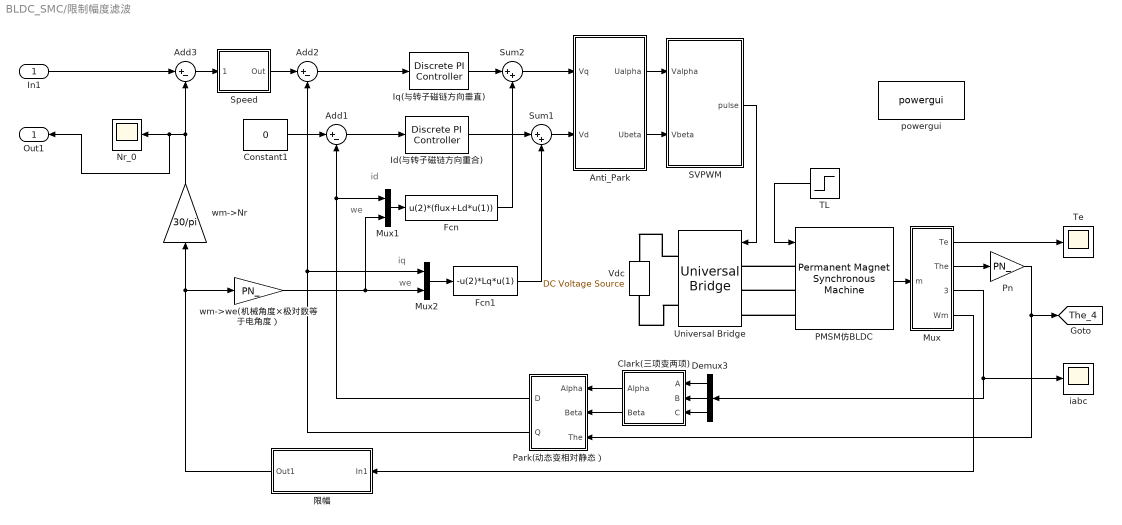
== system BLDC_SMC/限制幅度滤波 ==
  note: iq
  note: we
  note: we
  note: id
  In1 : Inport
  Add1 : Sum  Inputs=|+-
  Add2 : Sum  Inputs=|+-
  Add3 : Sum  Inputs=|+-
  Anti_Park : Subsystem
  Clark(三项变两项) : Subsystem
  Constant1 : Constant  Value=0
  Demux3 : Demux  Outputs=3
  Fcn : Fcn  Expr=u(2)*(flux+Ld*u(1))
  Fcn1 : Fcn  Expr=-u(2)*Lq*u(1)
  Id(与转子磁链方向重合) : powerlib_extras/Discrete  Control Blocks/Discrete PI Controller  Kp=Ld*2000  Ki=RS*2000  Par_Limits=[311*0.9*sqrt(1/3) -311*0.9*sqrt(1/3)]  Init=0  Ts=TS_1
  Iq(与转子磁链方向垂直) : powerlib_extras/Discrete  Control Blocks/Discrete PI Controller  Kp=Lq*2000  Ki=RS*2000  Par_Limits=[311*0.9*sqrt(1/3) -311*0.9*sqrt(1/3)]  Init=0  Ts=TS_1
  Mux : Subsystem
  Mux1 : Mux  Inputs=2
  Mux2 : Mux  Inputs=2
  Nr_0 : Scope
  PMSM仿BLDC : spsPermanentMagnetSynchronousMachineLib/Permanent Magnet Synchronous Machine  NbPhases=3  FluxDistribution=Sinusoidal  RotorType=Salient-pole  MechanicalLoad=Torque Tm  PresetModel=No  ShowDetailedParameters=on  MeasurementBus=off  Resistance=RS  Inductance=8.5e-3  dqInductances=LDLQ  La=0.000835  MachineConstant=Flux linkage established by magnets (V.s)  Flux=0.175  VoltageCst=222.1904  TorqueCst=1.8375  Flat=120  Mechanical=[0.003 0.008 7 0]  PolePairs=3  InitialConditions=[0,0, 0,0]  InitialConditions5ph=[0 0 0 0 0 0]  RefAngle=Aligned with phase A axis (original Park)  IterativeDiscreteModel=Trapezoidal non iterative  TsBlock=-1  TsPowergui=0
  Park(动态变相对静态） : Subsystem
  Pn : Gain  Gain=PN_
  SVPWM : Subsystem
  Speed : Subsystem  AncestorBlock=|  DialogController=POWERSYS.PowerSysDialog  mask(Discrete PI Controller){C=60, Mu=200, q=300, Par_Limits=[30 -30], Init=0, Ts=TS_1}
      | powerlib_extras/Discrete 
      | Control Blocks/Discrete
      | PI Controller
      mask prompts: C "Gain (c):"; Mu "Gain (Mu):"; q "Gain (q)"; Par_Limits "Output limits: [ Upper   Lower ]"; Init "Output initial value:"; Ts "Sample time:"
      mask help: This block implements a discrete PI controller.
      mask init:
      | UpperLimit=Par_Limits(1);
      | LowerLimit=Par_Limits(2);
      | power_initmask();
      mask Help: This block is part of a subset of blocks in the Extras library that does not have documentation associated with it, other than the block mask description.
      mask Display: disp('SMC');
  Sum1 : Sum  Inputs=|++
  Sum2 : Sum  Inputs=|++
  TL : Step  Time=0.2  After=10  SampleTime=0
  Te : Scope
  Universal Bridge : spsUniversalBridgeLib/Universal Bridge  Arms=3  SnubberResistance=1e5  SnubberCapacitance=inf  Device=IGBT / Diodes  Ron=1e-3  Lon=0  ForwardVoltages="[  0  0  ]"  ForwardVoltage=0  GTOparameters=[ 10e-6 , 20e-6 ]  IGBTparameters=[ 1e-6 , 2e-6 ]  Measurements=None  Measurements_2=None  converterType=Rectifier
  Vdc : spsDCVoltageSourceLib/DC Voltage Source  Amplitude=311  Measurements=None
  iabc : Scope
  powergui : sps_lib/powergui  SimulationMode=Continuous  SampleTime=Ts  frequency=60  Iterations=50  frequencyindice=0  Pbase=100e6  ErrMax=1e-4  UnitsV=kV  UnitsW=MW  buscounter=0  FunctionMessages=off  echomessages=off  EnableUseOfTLC=off  CurrentSourceSwitches=on  DisableSnubberDevices=off  DisableRonSwitches=off  DisableVfSwitches=off  DisplayEquations=off  AutomaticDiscreteSolvers=off  SolverType=Tustin/Backward Euler (TBE)  Interpol=off  ExternalGateDelay=off  methode=off  Ts=0  x0status=blocks  SPID=off  SwTol=0  HookPort=off  NonlinearTolerance=1e-4  nMaxIteration=100  ContinueOnMaxIteration=off  RestoreLinks=warning  ResistiveCurrentMeasurement=off  Frange=[0:2:500]  Ylog=off  Xlog=on  ShowGrid=off  save=off  variable=ZData  structure=0  ZoomFFT=on  StartTime=0.0  cycles=1  DisplayStyle=1  fundamental=60  FreqAxis=off  MaxFrequency=1000  frequencyindicesteady=1  RmsSteady=1  display=off
  wm->Nr : Gain  Gain=30/pi
  wm->we(机械角度×极对数等于电角度） : Gain  Gain=PN_
  限幅 : Subsystem
  Out1 : Outport
  tag scope: The_4=global
  wires:
  Pn/1 -> Park(动态变相对静态）/3(The), [The_4]
  SVPWM/1(pulse) -> Universal Bridge/1
  Add1/1 -> Id(与转子磁链方向重合)/1
  In1/1 -> Add3/1
  Fcn/1 -> Sum2/2
  Id(与转子磁链方向重合)/1 -> Sum1/1
  Mux2/1 -> Fcn1/1
  wm->Nr/1 -> Add3/2, Out1/1, Nr_0/1
  Clark(三项变两项)/2(Beta) -> Park(动态变相对静态）/2(Beta)
  Iq(与转子磁链方向垂直)/1 -> Sum2/1
  Sum2/1 -> Anti_Park/1(Vq)
  Speed/1(Out) -> Add2/1
  Add2/1 -> Iq(与转子磁链方向垂直)/1
  Fcn1/1 -> Sum1/2
  Park(动态变相对静态）/2(Q) -> Mux2/1, Add2/2
  Mux/4(Wm) -> 限幅/1(In1)
  Constant1/1 -> Add1/1
  Sum1/1 -> Anti_Park/2(Vd)
  Add3/1 -> Speed/1(Error)
  Mux/1(Te) -> Te/1
  Mux/2(The) -> Pn/1
  Anti_Park/2(Ubeta) -> SVPWM/2(Vbeta)
  Demux3/1 -> Clark(三项变两项)/1(A)
  Demux3/3 -> Clark(三项变两项)/3(C)
  Mux/3(Iabc) -> iabc/1, Demux3/1
  Demux3/2 -> Clark(三项变两项)/2(B)
  Mux1/1 -> Fcn/1
  TL/1 -> PMSM仿BLDC/1
  PMSM仿BLDC/1 -> Mux/1(m)
  Clark(三项变两项)/1(Alpha) -> Park(动态变相对静态）/1(Alpha)
  Park(动态变相对静态）/1(D) -> Mux1/1, Add1/2
  Anti_Park/1(Ualpha) -> SVPWM/1(Valpha)
  wm->we(机械角度×极对数等于电角度）/1 -> Mux2/2, Mux1/2
  限幅/1(Out1) -> wm->we(机械角度×极对数等于电角度）/1, wm->Nr/1
  connections:
  PMSM仿BLDC/LConn2 -- Universal Bridge/LConn2
  Universal Bridge/RConn1 -- Vdc/RConn1
  PMSM仿BLDC/LConn1 -- Universal Bridge/LConn1
  PMSM仿BLDC/LConn3 -- Universal Bridge/LConn3
  Universal Bridge/RConn2 -- Vdc/LConn1

== system BLDC_SMC/限幅滤波 ==
  In1 : Inport
  Abs : Abs  SaturateOnIntegerOverflow=off
  Add : Sum  Inputs=+-
  Delay : Delay  DelayLength=1  InitialCondition=0
  Multiport Selector : dspindex/Multiport Selector  rowsOrCols=Rows  idxCellArray={ 4, [1:2 5], [7; 8], 10:-1:6 }  idxErrMode=Clip Index
  Switch : Switch  Criteria=u2 > Threshold  Threshold=0.5  SaturateOnIntegerOverflow=off  InputSameDT=off
  Out1 : Outport
  wires:
  In1/1 -> Switch/3, Add/1
  Delay/1 -> Switch/1, Add/2
  Add/1 -> Abs/1
  Abs/1 -> Switch/2
  Switch/1 -> Delay/1, Out1/1

== system BLDC_SMC/RC/Anti_Park ==
  Vq : Inport
  Vd : Inport  Port=2
  Fcn : Fcn  Expr=cos(u[1])*u[2]-sin(u[1])*u[3]
  Fcn1 : Fcn  Expr=sin(u[1])*u[2]+cos(u[1])*u[3]
  Mux1 : Mux  Inputs=3
  Ualpha : Outport
  Ubeta : Outport  Port=2
  wires:
  Fcn1/1 -> Ubeta/1
  Fcn/1 -> Ualpha/1
  Mux1/1 -> Fcn/1, Fcn1/1
  Vd/1 -> Mux1/2
  Vq/1 -> Mux1/3
  [The] -> Mux1/1

== system BLDC_SMC/RC/Clark ==
  A : Inport
  B : Inport  Port=2
  C : Inport  Port=3
  Mux : Mux  Inputs=3
  alpha : Fcn  Expr=(u(1)-0.5*(u(2)+u(3)))*2/3
  beta : Fcn  Expr=sqrt(3)/2*(u(2)-u(3))*2/3
  Alpha : Outport
  Beta : Outport  Port=2
  wires:
  alpha/1 -> Alpha/1
  B/1 -> Mux/2
  C/1 -> Mux/3
  A/1 -> Mux/1
  Mux/1 -> beta/1, alpha/1
  beta/1 -> Beta/1

== system BLDC_SMC/RC/Mux ==
  m : Inport
  Bus Selector : BusSelector  OutputSignals=Stator current is_a (A),Stator current is_b (A),Stator current is_c (A)
  Bus Selector1 : BusSelector  OutputSignals=Rotor speed wm (rad/s),Rotor angle thetam (rad),Electromagnetic torque Te (N*m)
  Mux : Mux  Inputs=3
  Te : Outport
  The : Outport  Port=2
  Iabc : Outport  Port=3
  Wm : Outport  Port=4
  wires:
  Bus Selector1/1 -> Wm/1  "<Rotor speed wm (rad/s)>"
  Bus Selector1/2 -> The/1  "<Rotor angle thetam (rad)>"
  Bus Selector1/3 -> Te/1  "<Electromagnetic torque Te (N*m)>"
  m/1 -> Bus Selector/1, Bus Selector1/1
  Bus Selector/2 -> Mux/2  "<Stator current is_b (A)>"
  Bus Selector/3 -> Mux/3  "<Stator current is_c (A)>"
  Bus Selector/1 -> Mux/1  "<Stator current is_a (A)>"
  Mux/1 -> Iabc/1

== system BLDC_SMC/RC/Park ==
  Alpha : Inport
  Beta : Inport  Port=2
  The : Inport  Port=3
  Mux : Mux  Inputs=3
  d : Fcn  Expr=u(1)*cos(u(3))+u(2)*sin(u(3))
  q : Fcn  Expr=-u(1)*sin(u(3))+u(2)*cos(u(3))
  D : Outport
  Q : Outport  Port=2
  wires:
  d/1 -> D/1
  Beta/1 -> Mux/2
  The/1 -> Mux/3
  Alpha/1 -> Mux/1
  Mux/1 -> q/1, d/1
  q/1 -> Q/1

== system BLDC_SMC/RC/RC滤波 ==
  Wm : Inport
  α : Inport  Port=2
  Add : Sum  Inputs=-+
  Add2 : Sum
  Constant : Constant
  Delay : Delay  DelayLength=1  InitialCondition=0
  Product : Product
  Product1 : Product
  Out1 : Outport
  wires:
  Wm/1 -> Product/1
  α/1 -> Add/1, Product/2
  Constant/1 -> Add/2
  Product/1 -> Add2/1
  Add2/1 -> Delay/1, Out1/1
  Add/1 -> Product1/1
  Product1/1 -> Add2/2
  Delay/1 -> Product1/2

== system BLDC_SMC/RC/SVPWM ==
  Valpha : Inport
  Vbeta : Inport  Port=2
  PWM : Subsystem
  Repeating Sequence : simulink/Sources/Repeating Sequence  rep_seq_t=[0 0.00005 0.0001]  rep_seq_y=[0 0.00005 0]
  Sector Caculate : Subsystem
  T1T1 Caculate : Subsystem
  Tcm Caculate : Subsystem
  Tpwm : Constant  Value=0.0001
  Vdc : Constant  Value=311
  XYZ Caculate : Subsystem
  pulse : Outport
  wires:
  PWM/1(PWM) -> pulse/1
  Repeating Sequence/1 -> PWM/1(In)
  Vbeta/1 -> XYZ Caculate/2(Ubeta), Sector Caculate/2(Ubeta)
  T1T1 Caculate/1(T1) -> Tcm Caculate/2(T1)
  Valpha/1 -> XYZ Caculate/1(Ualpha), Sector Caculate/1(Ualpha)
  T1T1 Caculate/2(T2) -> Tcm Caculate/3(T2)
  Sector Caculate/1("N ") -> Tcm Caculate/1(N), T1T1 Caculate/1(N)
  XYZ Caculate/1(XYZ) -> T1T1 Caculate/2(XYZ)
  Tpwm/1 -> XYZ Caculate/3(Ts), Tcm Caculate/4(Tpwm), T1T1 Caculate/3(Tpwm)
  Vdc/1 -> XYZ Caculate/4(Udc)
  Tcm Caculate/1(Tcm1 Tcm2 Tcm3) -> PWM/2(Tcm123)

== system BLDC_SMC/RC/Speed ==
  Error : Inport  SampleTime=Ts
  1/D : Gain  Gain=1/(1.5*Pn*flux/0.003)  SaturateOnIntegerOverflow=on  SampleTime=Ts  OutDataTypeStr=Inherit: Same as input  ParamDataTypeStr=Inherit: Same as input
  Discrete Derivative : simulink/Discrete/Discrete Derivative  gainval=1.0  ICPrevScaledInput=0.0  OutMin=[]  OutMax=[]  OutDataType=fixdt(1, 16)  OutScaling=2^-10  DoSatur=off
  Discrete-Time Integrator : DiscreteIntegrator  InitialCondition=0.001  SampleTime=Ts  ICPrevOutput=DiscIntNeverNeededParam  ICPrevScaledInput=DiscIntNeverNeededParam
  Kp1 : Gain  Gain=q  SaturateOnIntegerOverflow=on  SampleTime=Ts  OutDataTypeStr=Inherit: Same as input  ParamDataTypeStr=Inherit: Same as input
  Kp2 : Gain  Gain=Mu  SaturateOnIntegerOverflow=on  SampleTime=Ts  OutDataTypeStr=Inherit: Same as input  ParamDataTypeStr=Inherit: Same as input
  Kp3 : Gain  Gain=C  SaturateOnIntegerOverflow=on  SampleTime=Ts  OutDataTypeStr=Inherit: Same as input  ParamDataTypeStr=Inherit: Same as input
  Kp4 : Gain  Gain=C  SaturateOnIntegerOverflow=on  SampleTime=Ts  OutDataTypeStr=Inherit: Same as input  ParamDataTypeStr=Inherit: Same as input
  Nr->wm : Gain  Gain=pi/30  SaturateOnIntegerOverflow=on  SampleTime=Ts  OutDataTypeStr=Inherit: Same as input  ParamDataTypeStr=Inherit: Same as input
  Saturation2 : Saturate  UpperLimit=UpperLimit  LowerLimit=LowerLimit  SampleTime=Ts
  Sign : Signum
  Sum1 : Sum  InputSameDT=on  SaturateOnIntegerOverflow=on  SampleTime=Ts  OutDataTypeStr=Inherit: Same as first input
  Sum2 : Sum  Inputs=+++  InputSameDT=on  SaturateOnIntegerOverflow=on  SampleTime=Ts  OutDataTypeStr=Inherit: Same as first input
  Out : Outport  SampleTime=Ts  InitialOutput=0
  wires:
  Kp4/1 -> Sum1/1
  Saturation2/1 -> Out/1
  Discrete Derivative/1 -> Kp3/1, Sum1/2
  Sum2/1 -> Discrete-Time Integrator/1
  Error/1 -> Nr->wm/1
  Kp1/1 -> Sum2/1
  Sign/1 -> Kp2/1
  Sum1/1 -> Sign/1, Kp1/1
  Kp2/1 -> Sum2/2
  Kp3/1 -> Sum2/3
  1/D/1 -> Saturation2/1
  Discrete-Time Integrator/1 -> 1/D/1
  Nr->wm/1 -> Discrete Derivative/1, Kp4/1

== system BLDC_SMC/中值滤波/Anti_Park ==
  Vq : Inport
  Vd : Inport  Port=2
  Fcn : Fcn  Expr=cos(u[1])*u[2]-sin(u[1])*u[3]
  Fcn1 : Fcn  Expr=sin(u[1])*u[2]+cos(u[1])*u[3]
  Mux1 : Mux  Inputs=3
  Ualpha : Outport
  Ubeta : Outport  Port=2
  wires:
  Fcn1/1 -> Ubeta/1
  Fcn/1 -> Ualpha/1
  Mux1/1 -> Fcn/1, Fcn1/1
  Vd/1 -> Mux1/2
  Vq/1 -> Mux1/3
  [The_3] -> Mux1/1

== system BLDC_SMC/中值滤波/Clark(三项变两项) ==
  A : Inport
  B : Inport  Port=2
  C : Inport  Port=3
  Mux : Mux  Inputs=3
  alpha : Fcn  Expr=(u(1)-0.5*(u(2)+u(3)))*2/3
  beta : Fcn  Expr=sqrt(3)/2*(u(2)-u(3))*2/3
  Alpha : Outport
  Beta : Outport  Port=2
  wires:
  alpha/1 -> Alpha/1
  B/1 -> Mux/2
  C/1 -> Mux/3
  A/1 -> Mux/1
  Mux/1 -> beta/1, alpha/1
  beta/1 -> Beta/1

== system BLDC_SMC/中值滤波/Mux ==
  m : Inport
  Bus Selector : BusSelector  OutputSignals=Stator current is_a (A),Stator current is_b (A),Stator current is_c (A)
  Bus Selector1 : BusSelector  OutputSignals=Rotor speed wm (rad/s),Rotor angle thetam (rad),Electromagnetic torque Te (N*m)
  Mux : Mux  Inputs=3
  Te : Outport
  The : Outport  Port=2
  Iabc : Outport  Port=3
  Wm : Outport  Port=4
  wires:
  Bus Selector1/1 -> Wm/1  "<Rotor speed wm (rad/s)>"
  Bus Selector1/2 -> The/1  "<Rotor angle thetam (rad)>"
  Bus Selector1/3 -> Te/1  "<Electromagnetic torque Te (N*m)>"
  m/1 -> Bus Selector/1, Bus Selector1/1
  Bus Selector/2 -> Mux/2  "<Stator current is_b (A)>"
  Bus Selector/3 -> Mux/3  "<Stator current is_c (A)>"
  Bus Selector/1 -> Mux/1  "<Stator current is_a (A)>"
  Mux/1 -> Iabc/1

== system BLDC_SMC/中值滤波/Park(动态变相对静态） ==
  Alpha : Inport
  Beta : Inport  Port=2
  The : Inport  Port=3
  Mux : Mux  Inputs=3
  d : Fcn  Expr=u(1)*cos(u(3))+u(2)*sin(u(3))
  q : Fcn  Expr=-u(1)*sin(u(3))+u(2)*cos(u(3))
  D : Outport
  Q : Outport  Port=2
  wires:
  d/1 -> D/1
  Beta/1 -> Mux/2
  The/1 -> Mux/3
  Alpha/1 -> Mux/1
  Mux/1 -> q/1, d/1
  q/1 -> Q/1

== system BLDC_SMC/中值滤波/SVPWM ==
  Valpha : Inport
  Vbeta : Inport  Port=2
  PWM : Subsystem
  Repeating Sequence : simulink/Sources/Repeating Sequence  rep_seq_t=[0 0.00005 0.0001]  rep_seq_y=[0 0.00005 0]
  Sector Caculate : Subsystem
  T1T2 Caculate : Subsystem
  Tcm Caculate : Subsystem
  Tpwm : Constant  Value=0.0001
  Vdc : Constant  Value=311
  XYZ Caculate : Subsystem
  pulse : Outport
  wires:
  PWM/1(PWM) -> pulse/1
  Repeating Sequence/1 -> PWM/1(In)
  Vbeta/1 -> XYZ Caculate/2(Ubeta), Sector Caculate/2(Ubeta)
  T1T2 Caculate/1(T1) -> Tcm Caculate/2(T1)
  Valpha/1 -> XYZ Caculate/1(Ualpha), Sector Caculate/1(Ualpha)
  T1T2 Caculate/2(T2) -> Tcm Caculate/3(T2)
  Sector Caculate/1("N ") -> Tcm Caculate/1(N), T1T2 Caculate/1(N)
  XYZ Caculate/1(XYZ) -> T1T2 Caculate/2(XYZ)
  Tpwm/1 -> XYZ Caculate/3(Ts), Tcm Caculate/4(Tpwm), T1T2 Caculate/3(Tpwm)
  Vdc/1 -> XYZ Caculate/4(Udc)
  Tcm Caculate/1(Tcm1 Tcm2 Tcm3) -> PWM/2(Tcm123)

== system BLDC_SMC/中值滤波/Speed ==
  Error : Inport  SampleTime=Ts
  1/D : Gain  Gain=1/(1.5*Pn*flux/0.003)  SaturateOnIntegerOverflow=on  SampleTime=Ts  OutDataTypeStr=Inherit: Same as input  ParamDataTypeStr=Inherit: Same as input
  Discrete Derivative : simulink/Discrete/Discrete Derivative  gainval=1.0  ICPrevScaledInput=0.0  OutMin=[]  OutMax=[]  OutDataType=fixdt(1, 16)  OutScaling=2^-10  DoSatur=off
  Discrete-Time Integrator : DiscreteIntegrator  InitialCondition=0.001  SampleTime=Ts  ICPrevOutput=DiscIntNeverNeededParam  ICPrevScaledInput=DiscIntNeverNeededParam
  Kp1 : Gain  Gain=q  SaturateOnIntegerOverflow=on  SampleTime=Ts  OutDataTypeStr=Inherit: Same as input  ParamDataTypeStr=Inherit: Same as input
  Kp2 : Gain  Gain=Mu  SaturateOnIntegerOverflow=on  SampleTime=Ts  OutDataTypeStr=Inherit: Same as input  ParamDataTypeStr=Inherit: Same as input
  Kp3 : Gain  Gain=C  SaturateOnIntegerOverflow=on  SampleTime=Ts  OutDataTypeStr=Inherit: Same as input  ParamDataTypeStr=Inherit: Same as input
  Kp4 : Gain  Gain=C  SaturateOnIntegerOverflow=on  SampleTime=Ts  OutDataTypeStr=Inherit: Same as input  ParamDataTypeStr=Inherit: Same as input
  Nr->wm : Gain  Gain=pi/30  SaturateOnIntegerOverflow=on  SampleTime=Ts  OutDataTypeStr=Inherit: Same as input  ParamDataTypeStr=Inherit: Same as input
  Saturation2 : Saturate  UpperLimit=UpperLimit  LowerLimit=LowerLimit  SampleTime=Ts
  Sign : Signum
  Sum1 : Sum  InputSameDT=on  SaturateOnIntegerOverflow=on  SampleTime=Ts  OutDataTypeStr=Inherit: Same as first input
  Sum2 : Sum  Inputs=+++  InputSameDT=on  SaturateOnIntegerOverflow=on  SampleTime=Ts  OutDataTypeStr=Inherit: Same as first input
  Out : Outport  SampleTime=Ts  InitialOutput=0
  wires:
  Kp4/1 -> Sum1/1
  Saturation2/1 -> Out/1
  Discrete Derivative/1 -> Kp3/1, Sum1/2
  Sum2/1 -> Discrete-Time Integrator/1
  Error/1 -> Nr->wm/1
  Kp1/1 -> Sum2/1
  Sign/1 -> Kp2/1
  Sum1/1 -> Sign/1, Kp1/1
  Kp2/1 -> Sum2/2
  Kp3/1 -> Sum2/3
  1/D/1 -> Saturation2/1
  Discrete-Time Integrator/1 -> 1/D/1
  Nr->wm/1 -> Discrete Derivative/1, Kp4/1

== system BLDC_SMC/控制IIR/Anti_Park ==
  Vq : Inport
  Vd : Inport  Port=2
  Fcn : Fcn  Expr=cos(u[1])*u[2]-sin(u[1])*u[3]
  Fcn1 : Fcn  Expr=sin(u[1])*u[2]+cos(u[1])*u[3]
  Mux1 : Mux  Inputs=3
  Ualpha : Outport
  Ubeta : Outport  Port=2
  wires:
  Fcn1/1 -> Ubeta/1
  Fcn/1 -> Ualpha/1
  Mux1/1 -> Fcn/1, Fcn1/1
  Vd/1 -> Mux1/2
  Vq/1 -> Mux1/3
  [The_2] -> Mux1/1

== system BLDC_SMC/控制IIR/Clark(三项变两项) ==
  A : Inport
  B : Inport  Port=2
  C : Inport  Port=3
  Mux : Mux  Inputs=3
  alpha : Fcn  Expr=(u(1)-0.5*(u(2)+u(3)))*2/3
  beta : Fcn  Expr=sqrt(3)/2*(u(2)-u(3))*2/3
  Alpha : Outport
  Beta : Outport  Port=2
  wires:
  alpha/1 -> Alpha/1
  B/1 -> Mux/2
  C/1 -> Mux/3
  A/1 -> Mux/1
  Mux/1 -> beta/1, alpha/1
  beta/1 -> Beta/1

== system BLDC_SMC/控制IIR/Mux ==
  m : Inport
  Bus Selector : BusSelector  OutputSignals=Stator current is_a (A),Stator current is_b (A),Stator current is_c (A)
  Bus Selector1 : BusSelector  OutputSignals=Rotor speed wm (rad/s),Rotor angle thetam (rad),Electromagnetic torque Te (N*m)
  Mux : Mux  Inputs=3
  Te : Outport
  The : Outport  Port=2
  Iabc : Outport  Port=3
  Wm : Outport  Port=4
  wires:
  Bus Selector1/1 -> Wm/1  "<Rotor speed wm (rad/s)>"
  Bus Selector1/2 -> The/1  "<Rotor angle thetam (rad)>"
  Bus Selector1/3 -> Te/1  "<Electromagnetic torque Te (N*m)>"
  m/1 -> Bus Selector/1, Bus Selector1/1
  Bus Selector/2 -> Mux/2  "<Stator current is_b (A)>"
  Bus Selector/3 -> Mux/3  "<Stator current is_c (A)>"
  Bus Selector/1 -> Mux/1  "<Stator current is_a (A)>"
  Mux/1 -> Iabc/1

== system BLDC_SMC/控制IIR/Park(动态变相对静态） ==
  Alpha : Inport
  Beta : Inport  Port=2
  The : Inport  Port=3
  Mux : Mux  Inputs=3
  d : Fcn  Expr=u(1)*cos(u(3))+u(2)*sin(u(3))
  q : Fcn  Expr=-u(1)*sin(u(3))+u(2)*cos(u(3))
  D : Outport
  Q : Outport  Port=2
  wires:
  d/1 -> D/1
  Beta/1 -> Mux/2
  The/1 -> Mux/3
  Alpha/1 -> Mux/1
  Mux/1 -> q/1, d/1
  q/1 -> Q/1

== system BLDC_SMC/控制IIR/SVPWM ==
  Valpha : Inport
  Vbeta : Inport  Port=2
  PWM : Subsystem
  Repeating Sequence : simulink/Sources/Repeating Sequence  rep_seq_t=[0 0.00005 0.0001]  rep_seq_y=[0 0.00005 0]
  Sector Caculate : Subsystem
  T1T2 Caculate : Subsystem
  Tcm Caculate : Subsystem
  Tpwm : Constant  Value=0.0001
  Vdc : Constant  Value=311
  XYZ Caculate : Subsystem
  pulse : Outport
  wires:
  PWM/1(PWM) -> pulse/1
  Repeating Sequence/1 -> PWM/1(In)
  Vbeta/1 -> XYZ Caculate/2(Ubeta), Sector Caculate/2(Ubeta)
  T1T2 Caculate/1(T1) -> Tcm Caculate/2(T1)
  Valpha/1 -> XYZ Caculate/1(Ualpha), Sector Caculate/1(Ualpha)
  T1T2 Caculate/2(T2) -> Tcm Caculate/3(T2)
  Sector Caculate/1("N ") -> Tcm Caculate/1(N), T1T2 Caculate/1(N)
  XYZ Caculate/1(XYZ) -> T1T2 Caculate/2(XYZ)
  Tpwm/1 -> XYZ Caculate/3(Ts), Tcm Caculate/4(Tpwm), T1T2 Caculate/3(Tpwm)
  Vdc/1 -> XYZ Caculate/4(Udc)
  Tcm Caculate/1(Tcm1 Tcm2 Tcm3) -> PWM/2(Tcm123)
